simulink model "octocopter_control_flow"  (R2024a)
settings: Solver=FixedStepAuto  StartTime=0.0  StopTime=inf
model workspace (MAT data in the model file):
  Ixx_values = 1.545e-05
  Iyy_values = 0.00073574
  Izz_values = 0.00074861
  base_link_Ixx = 7.46
  base_link_Iyy = 1.52
  base_link_Izz = 8.88
  base_link_mass = 19.0939
  gps0_Ixx = 2.1733e-06
  gps0_Iyy = 2.1733e-06
  gps0_Izz = 1.8e-07
  gps0_mass = 0.01
  i = 8
  imu_link_Ixx = 1e-05
  imu_link_Iyy = 1e-05
  imu_link_Izz = 1e-05
  imu_link_mass = 0.015
  masses = 0.085251
  phi : object (value not decoded)
  rotors : object (value not decoded)
  theta : object (value not decoded)
  total_Ixx = 7.46
  total_Iyy = 1.53
  total_Izz = 8.89
  total_mass = 20
  total_rotor_Ixx = 0.0001236
  total_rotor_Iyy = 0.00588592
  total_rotor_Izz = 0.00598888
  total_rotor_masses = 0.682008
  u : object (value not decoded)
  v : object (value not decoded)
  w : object (value not decoded)
  x : object (value not decoded)
  y : object (value not decoded)
  z : object (value not decoded)
values from neighbouring files (symbols this model uses):
  err1Enable = 0    [drone_6dof.m]    (also in octocopter_model_for_agressive.m; octocopter_model_for_orbit.m)
  err2Enable = 0    [drone_6dof.m]    (also in octocopter_model_for_agressive.m; octocopter_model_for_orbit.m)
  err3Enable = 0    [drone_6dof.m]    (also in octocopter_model_for_agressive.m; octocopter_model_for_orbit.m)
  err4Enable = 0    [drone_6dof.m]    (also in octocopter_model_for_agressive.m; octocopter_model_for_orbit.m)
  err5Enable = 0    [drone_6dof.m]    (also in octocopter_model_for_agressive.m; octocopter_model_for_orbit.m)
  err6Enable = 0    [drone_6dof.m]    (also in octocopter_model_for_agressive.m; octocopter_model_for_orbit.m)
  err7Enable = 0    [drone_6dof.m]    (also in octocopter_model_for_agressive.m; octocopter_model_for_orbit.m)
  err8Enable = 0    [drone_6dof.m]    (also in octocopter_model_for_agressive.m; octocopter_model_for_orbit.m)
  EulerInt_initial = [0;0;0]    [drone_6dof.m]    (also in octocopter_model_for_agressive.m; octocopter_model_for_orbit.m)
  motorErr1Time = 0    [drone_6dof.m]    (also in octocopter_model_for_agressive.m; octocopter_model_for_orbit.m)
  motorErr2Time = 0    [drone_6dof.m]    (also in octocopter_model_for_agressive.m; octocopter_model_for_orbit.m)
  motorErr3Time = 0    [drone_6dof.m]    (also in octocopter_model_for_agressive.m; octocopter_model_for_orbit.m)
  motorErr4Time = 0    [drone_6dof.m]    (also in octocopter_model_for_agressive.m; octocopter_model_for_orbit.m)
  motorErr5Time = 0    [drone_6dof.m]    (also in octocopter_model_for_agressive.m; octocopter_model_for_orbit.m)
  motorErr6Time = 0    [drone_6dof.m]    (also in octocopter_model_for_agressive.m; octocopter_model_for_orbit.m)
  motorErr7Time = 0    [drone_6dof.m]    (also in octocopter_model_for_agressive.m; octocopter_model_for_orbit.m)
  motorErr8Time = 0    [drone_6dof.m]    (also in octocopter_model_for_agressive.m; octocopter_model_for_orbit.m)
  omegaInt_initial = [0;0;0]    [drone_6dof.m]    (also in octocopter_model_for_agressive.m; octocopter_model_for_orbit.m)
  PosInertialInt_initial = [0;0;0]    [drone_6dof.m]    (also in octocopter_model_for_agressive.m; octocopter_model_for_orbit.m)
  vbInt_initial = [0;0;0]    [drone_6dof.m]    (also in octocopter_model_for_agressive.m; octocopter_model_for_orbit.m)
undefined symbols (not defined in the file or in its folder): DiscIntNeverNeededParam, PID_x_D, PID_x_I, PID_x_N, PID_y_D, PID_y_I, PID_y_N, PID_z_D, PID_z_I, PID_z_N, rad, rotor_max_rad_per_s, rotor_min_rad_per_s, s
libraries: robotlib x15, slpidlib x10, aerolibconvert2 x10, cstblocks x7, simulink x6, sharedtransform x4, dspmathops x1, vrlib x1, sharedutil x1, simulink_extras x1
(part 2 of 2)

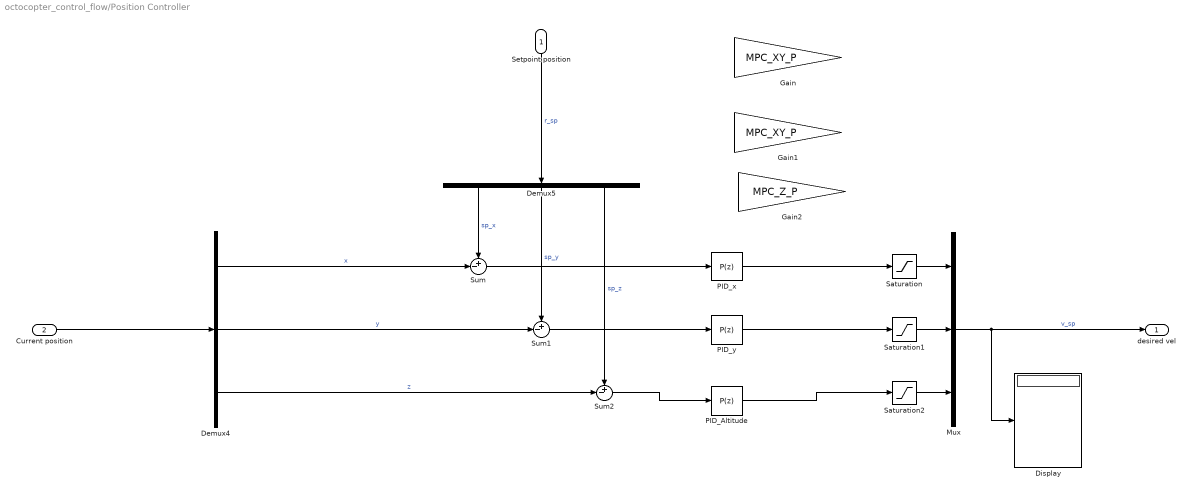
== system octocopter_control_flow/Position Controller ==
  Setpoint position : Inport
  Current position : Inport  Port=2
  Demux4 : Demux  Outputs=3
  Demux5 : Demux  Outputs=3
  Display : Display
  Gain : Gain  Gain=MPC_XY_P
  Gain1 : Gain  Gain=MPC_XY_P
  Gain2 : Gain  Gain=MPC_Z_P
  Mux : Mux  Inputs=3
  PID_Altitude : slpidlib/PID Controller  Controller=P  Form=Parallel  TimeDomain=Discrete-time  UseExternalTs=off  SampleTime=-1  IntegratorMethod=Backward Euler  FilterMethod=Forward Euler  ControllerParametersSource=internal  P=MPC_Z_P  I=PID_z_I  UseKiTs=off  D=PID_z_D  UseExternalDerivativeSource=off  N=PID_z_N  UseFilter=on  TunerSelectOption=Transfer Function Based (PID Tuner App)  InitialConditionSource=internal  InitialConditionForIntegrator=0  InitialConditionForFilter=0  DifferentiatorICPrevScaledInput=0  ExternalReset=level  TrackingMode=off  Kt=1  LimitOutput=on  SatLimitsSource=internal  UpperSaturationLimit=10  LowerSaturationLimit=-10  LinearizeAsGain=off  AntiWindupMode=clamping  Kb=1  LimitIntegrator=off  UpperIntegratorSaturationLimit=inf  LowerIntegratorSaturationLimit=-inf  POutMin=[]  POutMax=[]  IOutMin=[]  IOutMax=[]  DOutMin=[]  DOutMax=[]  NOutMin=[]  NOutMax=[]  SumOutMin=[]  SumOutMax=[]  SaturationOutMin=[]  SaturationOutMax=[]  PParamMin=[]  PParamMax=[]  IParamMin=[]  IParamMax=[]  DParamMin=[]  DParamMax=[]  NParamMin=[]  NParamMax=[]  KbParamMin=[]  KbParamMax=[]  KtParamMin=[]  KtParamMax=[]  KbOutMin=[]  KbOutMax=[]  KtOutMin=[]  KtOutMax=[]  IntegratorOutMin=[]  IntegratorOutMax=[]  FilterOutMin=[]  FilterOutMax=[]  SumI1OutMin=[]  SumI1OutMax=[]  SumI2OutMin=[]  SumI2OutMax=[]  SumI3OutMin=[]  SumI3OutMax=[]  SumI4OutMin=[]  SumI4OutMax=[]  SumDOutMin=[]  SumDOutMax=[]  DifferentiatorOutMin=[]  DifferentiatorOutMax=[]  FilterDiffOutCoefMin=[]  FilterDiffOutCoefMax=[]  ReciprocalOutMin=[]  ReciprocalOutMax=[]  SumDenOutMin=[]  SumDenOutMax=[]  SumNumOutMin=[]  SumNumOutMax=[]  DivideOutMin=[]  DivideOutMax=[]  UdiffTsProdOutMin=[]  UdiffTsProdOutMax=[]  NTsProdOutMin=[]  NTsProdOutMax=[]  UintegralTsProdOutMin=[]  UintegralTsProdOutMax=[]  UngainTsProdOutMin=[]  UngainTsProdOutMax=[]  ClampingZeroOutDataTypeStr=Inherit: Inherit via back propagation  ClampingZeroOutMin=[]  ClampingZeroOutMax=[]  FilterDenConstantOutDataTypeStr=Inherit: Inherit via back propagation  FilterDenConstantOutMin=[]  FilterDenConstantOutMax=[]  PCopyOutDataTypeStr=Inherit: Inherit via back propagation  PCopyOutMin=[]  PCopyOutMax=[]  NCopyOutDataTypeStr=Inherit: Inherit via back propagation  NCopyOutMin=[]  NCopyOutMax=[]  IntegratorContinuousStateAttributes=''  IntegratorStateMustResolveToSignalObject=off  IntegratorRTWStateStorageClass=Auto  FilterContinuousStateAttributes=''  FilterStateMustResolveToSignalObject=off  FilterRTWStateStorageClass=Auto  ParallelPVariant=InternalParameters  IdealPVariant=Disabled  IVariant=Disabled  DVariant=Disabled  IntegratorVariant=Disabled  SatVariant=Enabled  AWVariant=Disabled  PCopyVariant=Disabled  TRVariant=Disabled  FdbkBlocksVariant=Forward  IdealPFdbkVariant=Disabled  SatFdbkVariant=Disabled  DerivativeFilterVariant=Disabled  NVariant=Disabled  NCopyVariant=Disabled_SignalSpec  FilterICVariant=Disabled  IntegratorICVariant=Disabled  ExternalResetVariant=Disabled  TRSumVariant=Passthrough  SumFdbkVariant=Disabled  SumVariant=Passthrough_P  TsampFilterVariant=InternalTs  TsampNgainVariant=Passthrough  TsampIntegralVariant=Disabled_SignalSpec  ExternalSaturationOutDataTypeStr=Inherit: Same as second input  DerivativeSourceVariant=Disabled
  PID_x : slpidlib/PID Controller  Controller=P  Form=Parallel  TimeDomain=Discrete-time  UseExternalTs=off  SampleTime=-1  IntegratorMethod=Forward Euler  FilterMethod=Forward Euler  ControllerParametersSource=internal  P=MPC_XY_P  I=PID_x_I  UseKiTs=off  D=PID_x_D  UseExternalDerivativeSource=off  N=PID_x_N  UseFilter=on  TunerSelectOption=Transfer Function Based (PID Tuner App)  InitialConditionSource=internal  InitialConditionForIntegrator=0  InitialConditionForFilter=0  DifferentiatorICPrevScaledInput=0  ExternalReset=level  TrackingMode=off  Kt=1  LimitOutput=on  SatLimitsSource=internal  UpperSaturationLimit=20  LowerSaturationLimit=-20  LinearizeAsGain=off  AntiWindupMode=clamping  Kb=1  LimitIntegrator=off  UpperIntegratorSaturationLimit=inf  LowerIntegratorSaturationLimit=-inf  POutMin=[]  POutMax=[]  IOutMin=[]  IOutMax=[]  DOutMin=[]  DOutMax=[]  NOutMin=[]  NOutMax=[]  SumOutMin=[]  SumOutMax=[]  SaturationOutMin=[]  SaturationOutMax=[]  PParamMin=[]  PParamMax=[]  IParamMin=[]  IParamMax=[]  DParamMin=[]  DParamMax=[]  NParamMin=[]  NParamMax=[]  KbParamMin=[]  KbParamMax=[]  KtParamMin=[]  KtParamMax=[]  KbOutMin=[]  KbOutMax=[]  KtOutMin=[]  KtOutMax=[]  IntegratorOutMin=[]  IntegratorOutMax=[]  FilterOutMin=[]  FilterOutMax=[]  SumI1OutMin=[]  SumI1OutMax=[]  SumI2OutMin=[]  SumI2OutMax=[]  SumI3OutMin=[]  SumI3OutMax=[]  SumI4OutMin=[]  SumI4OutMax=[]  SumDOutMin=[]  SumDOutMax=[]  DifferentiatorOutMin=[]  DifferentiatorOutMax=[]  FilterDiffOutCoefMin=[]  FilterDiffOutCoefMax=[]  ReciprocalOutMin=[]  ReciprocalOutMax=[]  SumDenOutMin=[]  SumDenOutMax=[]  SumNumOutMin=[]  SumNumOutMax=[]  DivideOutMin=[]  DivideOutMax=[]  UdiffTsProdOutMin=[]  UdiffTsProdOutMax=[]  NTsProdOutMin=[]  NTsProdOutMax=[]  UintegralTsProdOutMin=[]  UintegralTsProdOutMax=[]  UngainTsProdOutMin=[]  UngainTsProdOutMax=[]  ClampingZeroOutDataTypeStr=Inherit: Inherit via back propagation  ClampingZeroOutMin=[]  ClampingZeroOutMax=[]  FilterDenConstantOutDataTypeStr=Inherit: Inherit via back propagation  FilterDenConstantOutMin=[]  FilterDenConstantOutMax=[]  PCopyOutDataTypeStr=Inherit: Inherit via back propagation  PCopyOutMin=[]  PCopyOutMax=[]  NCopyOutDataTypeStr=Inherit: Inherit via back propagation  NCopyOutMin=[]  NCopyOutMax=[]  IntegratorContinuousStateAttributes=''  IntegratorStateMustResolveToSignalObject=off  IntegratorRTWStateStorageClass=Auto  FilterContinuousStateAttributes=''  FilterStateMustResolveToSignalObject=off  FilterRTWStateStorageClass=Auto  ParallelPVariant=InternalParameters  IdealPVariant=Disabled  IVariant=Disabled  DVariant=Disabled  IntegratorVariant=Disabled  SatVariant=Enabled  AWVariant=Disabled  PCopyVariant=Disabled  TRVariant=Disabled  FdbkBlocksVariant=Forward  IdealPFdbkVariant=Disabled  SatFdbkVariant=Disabled  DerivativeFilterVariant=Disabled  NVariant=Disabled  NCopyVariant=Disabled_SignalSpec  FilterICVariant=Disabled  IntegratorICVariant=Disabled  ExternalResetVariant=Disabled  TRSumVariant=Passthrough  SumFdbkVariant=Disabled  SumVariant=Passthrough_P  TsampFilterVariant=InternalTs  TsampNgainVariant=Passthrough  TsampIntegralVariant=Disabled_SignalSpec  ExternalSaturationOutDataTypeStr=Inherit: Same as second input  DerivativeSourceVariant=Disabled
  PID_y : slpidlib/PID Controller  Controller=P  Form=Parallel  TimeDomain=Discrete-time  UseExternalTs=off  SampleTime=-1  IntegratorMethod=Forward Euler  FilterMethod=Forward Euler  ControllerParametersSource=internal  P=MPC_XY_P  I=PID_y_I  UseKiTs=off  D=PID_y_D  UseExternalDerivativeSource=off  N=PID_y_N  UseFilter=on  TunerSelectOption=Transfer Function Based (PID Tuner App)  InitialConditionSource=internal  InitialConditionForIntegrator=0  InitialConditionForFilter=0  DifferentiatorICPrevScaledInput=0  ExternalReset=level  TrackingMode=off  Kt=1  LimitOutput=on  SatLimitsSource=internal  UpperSaturationLimit=20  LowerSaturationLimit=-20  LinearizeAsGain=off  AntiWindupMode=clamping  Kb=1  LimitIntegrator=off  UpperIntegratorSaturationLimit=inf  LowerIntegratorSaturationLimit=-inf  POutMin=[]  POutMax=[]  IOutMin=[]  IOutMax=[]  DOutMin=[]  DOutMax=[]  NOutMin=[]  NOutMax=[]  SumOutMin=[]  SumOutMax=[]  SaturationOutMin=[]  SaturationOutMax=[]  PParamMin=[]  PParamMax=[]  IParamMin=[]  IParamMax=[]  DParamMin=[]  DParamMax=[]  NParamMin=[]  NParamMax=[]  KbParamMin=[]  KbParamMax=[]  KtParamMin=[]  KtParamMax=[]  KbOutMin=[]  KbOutMax=[]  KtOutMin=[]  KtOutMax=[]  IntegratorOutMin=[]  IntegratorOutMax=[]  FilterOutMin=[]  FilterOutMax=[]  SumI1OutMin=[]  SumI1OutMax=[]  SumI2OutMin=[]  SumI2OutMax=[]  SumI3OutMin=[]  SumI3OutMax=[]  SumI4OutMin=[]  SumI4OutMax=[]  SumDOutMin=[]  SumDOutMax=[]  DifferentiatorOutMin=[]  DifferentiatorOutMax=[]  FilterDiffOutCoefMin=[]  FilterDiffOutCoefMax=[]  ReciprocalOutMin=[]  ReciprocalOutMax=[]  SumDenOutMin=[]  SumDenOutMax=[]  SumNumOutMin=[]  SumNumOutMax=[]  DivideOutMin=[]  DivideOutMax=[]  UdiffTsProdOutMin=[]  UdiffTsProdOutMax=[]  NTsProdOutMin=[]  NTsProdOutMax=[]  UintegralTsProdOutMin=[]  UintegralTsProdOutMax=[]  UngainTsProdOutMin=[]  UngainTsProdOutMax=[]  ClampingZeroOutDataTypeStr=Inherit: Inherit via back propagation  ClampingZeroOutMin=[]  ClampingZeroOutMax=[]  FilterDenConstantOutDataTypeStr=Inherit: Inherit via back propagation  FilterDenConstantOutMin=[]  FilterDenConstantOutMax=[]  PCopyOutDataTypeStr=Inherit: Inherit via back propagation  PCopyOutMin=[]  PCopyOutMax=[]  NCopyOutDataTypeStr=Inherit: Inherit via back propagation  NCopyOutMin=[]  NCopyOutMax=[]  IntegratorContinuousStateAttributes=''  IntegratorStateMustResolveToSignalObject=off  IntegratorRTWStateStorageClass=Auto  FilterContinuousStateAttributes=''  FilterStateMustResolveToSignalObject=off  FilterRTWStateStorageClass=Auto  ParallelPVariant=InternalParameters  IdealPVariant=Disabled  IVariant=Disabled  DVariant=Disabled  IntegratorVariant=Disabled  SatVariant=Enabled  AWVariant=Disabled  PCopyVariant=Disabled  TRVariant=Disabled  FdbkBlocksVariant=Forward  IdealPFdbkVariant=Disabled  SatFdbkVariant=Disabled  DerivativeFilterVariant=Disabled  NVariant=Disabled  NCopyVariant=Disabled_SignalSpec  FilterICVariant=Disabled  IntegratorICVariant=Disabled  ExternalResetVariant=Disabled  TRSumVariant=Passthrough  SumFdbkVariant=Disabled  SumVariant=Passthrough_P  TsampFilterVariant=InternalTs  TsampNgainVariant=Passthrough  TsampIntegralVariant=Disabled_SignalSpec  ExternalSaturationOutDataTypeStr=Inherit: Same as second input  DerivativeSourceVariant=Disabled
  Saturation : Saturate  UpperLimit=MPC_XY_VEL_ALL  LowerLimit=-MPC_XY_VEL_ALL
  Saturation1 : Saturate  UpperLimit=MPC_XY_VEL_ALL  LowerLimit=-MPC_XY_VEL_ALL
  Saturation2 : Saturate  UpperLimit=1  LowerLimit=-1
  Sum : Sum  Inputs=+-|
  Sum1 : Sum  Inputs=+-|
  Sum2 : Sum  Inputs=+-|
  desired vel : Outport
  wires:
  Sum2/1 -> PID_Altitude/1
  Demux4/3 -> Sum2/2  "z"
  Current position/1 -> Demux4/1
  Saturation1/1 -> Mux/2
  Demux5/2 -> Sum1/1  "sp_y"
  Sum/1 -> PID_x/1
  Demux4/1 -> Sum/2  "x"
  PID_y/1 -> Saturation1/1
  Mux/1 -> desired vel/1, Display/1  "v_sp"
  Saturation2/1 -> Mux/3
  PID_x/1 -> Saturation/1
  PID_Altitude/1 -> Saturation2/1
  Demux5/1 -> Sum/1  "sp_x"
  Demux4/2 -> Sum1/2  "y"
  Demux5/3 -> Sum2/1  "sp_z"
  Saturation/1 -> Mux/1
  Setpoint position/1 -> Demux5/1  "r_sp"
  Sum1/1 -> PID_y/1

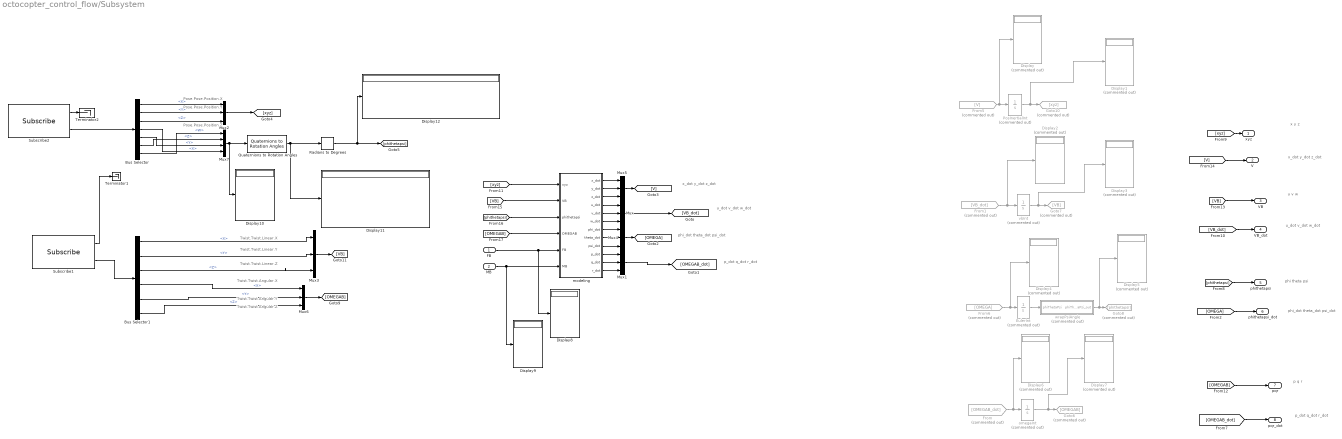
== system octocopter_control_flow/Subsystem ==
  note: Pose.Pose.Position.X
  note: x
      | y
      | z
  note: x_dot
      | y_dot
      | z_dot
  note: phi_dot
      | theta_dot
      | psi_dot
  note: phi
      | theta
      | psi
  note: p_dot
      | q_dot
      | r_dot
  note: p
      | q
      | r
  note: u
      | v
      | w
  note: u_dot
      | v_dot
      | w_dot
  note: x_dot
      | y_dot
      | z_dot
  note: u_dot
      | v_dot
      | w_dot
  note: phi_dot
      | theta_dot
      | psi_dot
  note: p_dot
      | q_dot
      | r_dot
  note: Pose.Pose.Position.Y
  note: Pose.Pose.Position.Z
  note: Twist.Twist.Linear.X
  note: Twist.Twist.Linear.Y
  note: Twist.Twist.Linear.Z
  note: Twist.Twist.Angular.X
  note: Twist.Twist.Angular.Y
  note: Twist.Twist.Angular.Z
  FB : Inport
  MB : Inport  Port=2
  Bus Selector : BusSelector  OutputSignals=Pose.Pose.Position.X,Pose.Pose.Position.Y,Pose.Pose.Position.Z,Pose.Pose.Orientation.X,Pose.Pose.Orientation.Y,Pose.Pose.Orientation.Z,Pose.Pose.Orientation.W
  Bus Selector1 : BusSelector  OutputSignals=Twist.Twist.Linear.X,Twist.Twist.Linear.Y,Twist.Twist.Linear.Z,Twist.Twist.Angular.X,Twist.Twist.Angular.Y,Twist.Twist.Angular.Z
  Display{,1..7} (8 alike) : Display  Commented=on
  Display{8..12} (5 alike) : Display
  EulerInt : Integrator  Commented=on  InitialCondition=EulerInt_initial
  From : From  Commented=on  GotoTag=OMEGAB_dot
  From1 : From  Commented=on  GotoTag=VB_dot
  From5 : From  Commented=on  GotoTag=V
  From6 : From  Commented=on  GotoTag=OMEGA
  Goto10 : Goto  Commented=on  GotoTag=xyz
  Goto6 : Goto  Commented=on  GotoTag=OMEGAB
  Goto7 : Goto  Commented=on  GotoTag=VB
  Goto8 : Goto  Commented=on  GotoTag=phithetapsi
  Mux{,1..6} (7 alike) : Mux  Inputs=3
  Mux7 : Mux
  PosInertialInt : Integrator  Commented=on  InitialCondition=PosInertialInt_initial
  Quaternions to Rotation Angles : sharedtransform/Quaternions to Rotation Angles  rotationOrder=ZYX  aMode=aMode
  Radians to Degrees : simulink_extras/Transformations/Radians to Degrees
  Subscribe1 : robotlib/Subscribe  topicSource=Select from ROS network  topic=/mavros/local_position/odom  messageType=nav_msgs/Odometry  SampleTime=-1  legacyBusStruct=off  messageQueueLength=1
  Subscribe2 : robotlib/Subscribe  topicSource=Select from ROS network  topic=/mavros/global_position/local  messageType=nav_msgs/Odometry  SampleTime=-1  legacyBusStruct=off  messageQueueLength=1
  Terminator1 : Terminator
  Terminator2 : Terminator
  modeling : MATLAB Function  TreatAsAtomicUnit=on
  omegaInt : Integrator  Commented=on  InitialCondition=omegaInt_initial  UpperSaturationLimit=rotor_max_rad_per_s  LowerSaturationLimit=rotor_min_rad_per_s
  vbInt : Integrator  Commented=on  InitialCondition=vbInt_initial
  wrapPsiAngle : Subsystem  Commented=on
  xyz : Outport
  V : Outport  Port=2
  VB : Outport  Port=3
  VB_dot : Outport  Port=4
  phithetapsi : Outport  Port=5
  phithetapsi_dot : Outport  Port=6
  pqr : Outport  Port=7
  pqr_dot : Outport  Port=8
  wires:
  From1/1 -> Display2/1, vbInt/1
  From5/1 -> Display/1, PosInertialInt/1
  EulerInt/1 -> wrapPsiAngle/1(phiThetaPsi)
  Mux1/1 -> [OMEGAB_dot]
  Mux4/1 -> [OMEGA]
  Mux/1 -> [VB_dot]
  PosInertialInt/1 -> Display1/1, Goto10/1
  Mux5/1 -> [V]
  omegaInt/1 -> Display7/1, Goto6/1
  modeling/11(q_dot) -> Mux1/2
  From6/1 -> Display4/1, EulerInt/1
  modeling/6(w_dot) -> Mux/3
  [V] -> V/1
  [xyz] -> xyz/1
  From/1 -> Display6/1, omegaInt/1
  modeling/3(z_dot) -> Mux5/3
  [phithetapsi] -> phithetapsi/1
  wrapPsiAngle/1(phiThetaPsi_out) -> Display5/1, Goto8/1
  modeling/4(u_dot) -> Mux/1
  modeling/8(theta_dot) -> Mux4/2
  modeling/5(v_dot) -> Mux/2
  modeling/12(r_dot) -> Mux1/3
  modeling/9(psi_dot) -> Mux4/3
  vbInt/1 -> Display3/1, Goto7/1
  modeling/7(phi_dot) -> Mux4/1
  modeling/2(y_dot) -> Mux5/2
  modeling/10(p_dot) -> Mux1/1
  modeling/1(x_dot) -> Mux5/1
  [OMEGA] -> phithetapsi_dot/1
  [OMEGAB_dot] -> pqr_dot/1
  [OMEGAB] -> pqr/1
  [VB_dot] -> VB_dot/1
  [VB] -> VB/1
  FB/1 -> Display8/1, modeling/5(FB)
  MB/1 -> Display9/1, modeling/6(MB)
  [OMEGAB] -> modeling/4(OMEGAB)
  [phithetapsi] -> modeling/3(phithetapsi)
  [VB] -> modeling/2(VB)
  [xyz] -> modeling/1(xyz)
  Bus Selector1/2 -> Mux3/2  "<Y>"
  Subscribe1/2 -> Bus Selector1/1
  Bus Selector1/4 -> Mux6/1  "<X>"
  Bus Selector1/1 -> Mux3/1  "<X>"
  Subscribe1/1 -> Terminator1/1
  Bus Selector1/3 -> Mux3/3  "<Z>"
  Bus Selector1/6 -> Mux6/3  "<Z>"
  Bus Selector1/5 -> Mux6/2  "<Y>"
  Mux2/1 -> [xyz]
  Mux6/1 -> [OMEGAB]
  Mux3/1 -> [VB]
  Subscribe2/2 -> Bus Selector/1
  Subscribe2/1 -> Terminator2/1
  Bus Selector/2 -> Mux2/2  "<Y>"
  Bus Selector/1 -> Mux2/1  "<X>"
  Bus Selector/3 -> Mux2/3  "<Z>"
  Mux7/1 -> Display10/1, Quaternions to Rotation Angles/1
  Quaternions to Rotation Angles/1 -> Display11/1, Radians to Degrees/1
  Bus Selector/7 -> Mux7/1  "<W>"
  Bus Selector/4 -> Mux7/4  "<X>"
  Bus Selector/5 -> Mux7/3  "<Y>"
  Bus Selector/6 -> Mux7/2  "<Z>"
  Radians to Degrees/1 -> Display12/1, [phithetapsi]

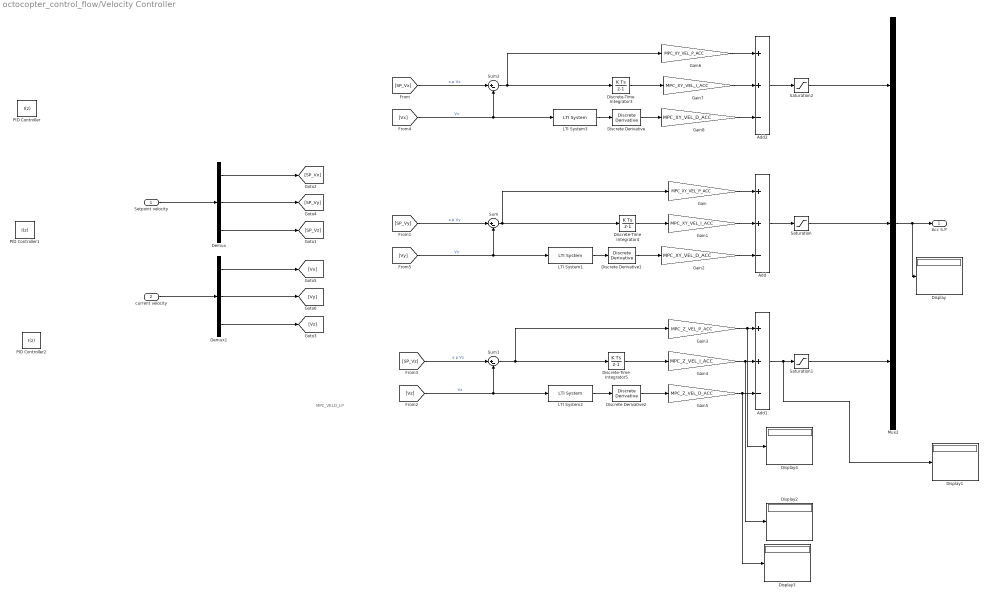
== system octocopter_control_flow/Velocity Controller ==
  note: MPC_VELD_LP
  Setpoint velocity : Inport
  current velocity : Inport  Port=2
  Add : Sum  Inputs=++-
  Add1 : Sum  Inputs=++-
  Add2 : Sum  Inputs=++-
  Demux : Demux  Outputs=3
  Demux1 : Demux  Outputs=3
  Discrete Derivative : simulink/Discrete/Discrete Derivative  gainval=1.0  ICPrevScaledInput=0.0  OutMin=[]  OutMax=[]  OutDataType=fixdt(1, 16)  OutScaling=2^-10  DoSatur=off
  Discrete Derivative1 : simulink/Discrete/Discrete Derivative  gainval=1.0  ICPrevScaledInput=0.0  OutMin=[]  OutMax=[]  OutDataType=fixdt(1, 16)  OutScaling=2^-10  DoSatur=off
  Discrete Derivative2 : simulink/Discrete/Discrete Derivative  gainval=1.0  ICPrevScaledInput=0.0  OutMin=[]  OutMax=[]  OutDataType=fixdt(1, 16)  OutScaling=2^-10  DoSatur=off
  Discrete-Time Integrator3 : DiscreteIntegrator  SampleTime=1/100  ICPrevOutput=DiscIntNeverNeededParam  ICPrevScaledInput=DiscIntNeverNeededParam
  Discrete-Time Integrator4 : DiscreteIntegrator  SampleTime=1/100  ICPrevOutput=DiscIntNeverNeededParam  ICPrevScaledInput=DiscIntNeverNeededParam
  Discrete-Time Integrator5 : DiscreteIntegrator  SampleTime=1/100  ICPrevOutput=DiscIntNeverNeededParam  ICPrevScaledInput=DiscIntNeverNeededParam
  Display{,1..4} (5 alike) : Display
  Gain : Gain  Gain=MPC_XY_VEL_P_ACC
  Gain1 : Gain  Gain=MPC_XY_VEL_I_ACC
  Gain2 : Gain  Gain=MPC_XY_VEL_D_ACC
  Gain3 : Gain  Gain=MPC_Z_VEL_P_ACC
  Gain4 : Gain  Gain=MPC_Z_VEL_I_ACC
  Gain5 : Gain  Gain=MPC_Z_VEL_D_ACC
  Gain6 : Gain  Gain=MPC_XY_VEL_P_ACC
  Gain7 : Gain  Gain=MPC_XY_VEL_I_ACC
  Gain8 : Gain  Gain=MPC_XY_VEL_D_ACC
  LTI System1 : cstblocks/LTI System  sys=c2d(tf(1,[MPC_VELD_LP 1]),1/100)  IC=[]  PadeOrder=0
  LTI System2 : cstblocks/LTI System  sys=c2d(tf(1,[MPC_VELD_LP 1]),1/100)  IC=[]  PadeOrder=0
  LTI System3 : cstblocks/LTI System  sys=c2d(tf(1,[MPC_VELD_LP 1]),1/100)  IC=[]  PadeOrder=0
  Mux2 : Mux  Inputs=3
  PID Controller : slpidlib/PID Controller  Controller=I  Form=Parallel  TimeDomain=Discrete-time  UseExternalTs=off  SampleTime=-1  IntegratorMethod=Forward Euler  FilterMethod=Forward Euler  ControllerParametersSource=internal  P=MPC_XY_VEL_P_ACC  I=MPC_XY_VEL_I_ACC  UseKiTs=off  D=0  UseExternalDerivativeSource=off  N=100  UseFilter=on  TunerSelectOption=Transfer Function Based (PID Tuner App)  InitialConditionSource=internal  InitialConditionForIntegrator=0  InitialConditionForFilter=0  DifferentiatorICPrevScaledInput=0  ExternalReset=none  TrackingMode=off  Kt=1  LimitOutput=on  SatLimitsSource=internal  UpperSaturationLimit=inf  LowerSaturationLimit=-inf  LinearizeAsGain=on  AntiWindupMode=clamping  Kb=1  LimitIntegrator=off  UpperIntegratorSaturationLimit=inf  LowerIntegratorSaturationLimit=-inf  POutMin=[]  POutMax=[]  IOutMin=[]  IOutMax=[]  DOutMin=[]  DOutMax=[]  NOutMin=[]  NOutMax=[]  SumOutMin=[]  SumOutMax=[]  SaturationOutMin=[]  SaturationOutMax=[]  PParamMin=[]  PParamMax=[]  IParamMin=[]  IParamMax=[]  DParamMin=[]  DParamMax=[]  NParamMin=[]  NParamMax=[]  KbParamMin=[]  KbParamMax=[]  KtParamMin=[]  KtParamMax=[]  KbOutMin=[]  KbOutMax=[]  KtOutMin=[]  KtOutMax=[]  IntegratorOutMin=[]  IntegratorOutMax=[]  FilterOutMin=[]  FilterOutMax=[]  SumI1OutMin=[]  SumI1OutMax=[]  SumI2OutMin=[]  SumI2OutMax=[]  SumI3OutMin=[]  SumI3OutMax=[]  SumI4OutMin=[]  SumI4OutMax=[]  SumDOutMin=[]  SumDOutMax=[]  DifferentiatorOutMin=[]  DifferentiatorOutMax=[]  FilterDiffOutCoefMin=[]  FilterDiffOutCoefMax=[]  ReciprocalOutMin=[]  ReciprocalOutMax=[]  SumDenOutMin=[]  SumDenOutMax=[]  SumNumOutMin=[]  SumNumOutMax=[]  DivideOutMin=[]  DivideOutMax=[]  UdiffTsProdOutMin=[]  UdiffTsProdOutMax=[]  NTsProdOutMin=[]  NTsProdOutMax=[]  UintegralTsProdOutMin=[]  UintegralTsProdOutMax=[]  UngainTsProdOutMin=[]  UngainTsProdOutMax=[]  ClampingZeroOutDataTypeStr=Inherit: Inherit via back propagation  ClampingZeroOutMin=[]  ClampingZeroOutMax=[]  FilterDenConstantOutDataTypeStr=Inherit: Inherit via back propagation  FilterDenConstantOutMin=[]  FilterDenConstantOutMax=[]  PCopyOutDataTypeStr=Inherit: Inherit via back propagation  PCopyOutMin=[]  PCopyOutMax=[]  NCopyOutDataTypeStr=Inherit: Inherit via back propagation  NCopyOutMin=[]  NCopyOutMax=[]  IntegratorContinuousStateAttributes=''  IntegratorStateMustResolveToSignalObject=off  IntegratorRTWStateStorageClass=Auto  FilterContinuousStateAttributes=''  FilterStateMustResolveToSignalObject=off  FilterRTWStateStorageClass=Auto  ParallelPVariant=Disabled  IdealPVariant=Disabled  IVariant=InternalParameters  DVariant=Disabled  IntegratorVariant=Discrete  SatVariant=Enabled  AWVariant=DiscClampingParallel  PCopyVariant=Disabled  TRVariant=Disabled  FdbkBlocksVariant=Forward  IdealPFdbkVariant=Disabled  SatFdbkVariant=Disabled  DerivativeFilterVariant=Disabled  NVariant=Disabled  NCopyVariant=Disabled_SignalSpec  FilterICVariant=Disabled  IntegratorICVariant=InternalICs  ExternalResetVariant=Disabled  TRSumVariant=Passthrough  SumFdbkVariant=Disabled  SumVariant=Passthrough_I  TsampFilterVariant=InternalTs  TsampNgainVariant=Passthrough  TsampIntegralVariant=Disabled_SignalSpec  ExternalSaturationOutDataTypeStr=Inherit: Same as second input  DerivativeSourceVariant=Disabled
  PID Controller1 : slpidlib/PID Controller  Controller=I  Form=Parallel  TimeDomain=Discrete-time  UseExternalTs=off  SampleTime=-1  IntegratorMethod=Forward Euler  FilterMethod=Forward Euler  ControllerParametersSource=internal  P=MPC_XY_VEL_P_ACC  I=MPC_XY_VEL_I_ACC  UseKiTs=off  D=0  UseExternalDerivativeSource=off  N=100  UseFilter=on  TunerSelectOption=Transfer Function Based (PID Tuner App)  InitialConditionSource=internal  InitialConditionForIntegrator=0  InitialConditionForFilter=0  DifferentiatorICPrevScaledInput=0  ExternalReset=none  TrackingMode=off  Kt=1  LimitOutput=on  SatLimitsSource=internal  UpperSaturationLimit=inf  LowerSaturationLimit=-inf  LinearizeAsGain=on  AntiWindupMode=clamping  Kb=1  LimitIntegrator=off  UpperIntegratorSaturationLimit=inf  LowerIntegratorSaturationLimit=-inf  POutMin=[]  POutMax=[]  IOutMin=[]  IOutMax=[]  DOutMin=[]  DOutMax=[]  NOutMin=[]  NOutMax=[]  SumOutMin=[]  SumOutMax=[]  SaturationOutMin=[]  SaturationOutMax=[]  PParamMin=[]  PParamMax=[]  IParamMin=[]  IParamMax=[]  DParamMin=[]  DParamMax=[]  NParamMin=[]  NParamMax=[]  KbParamMin=[]  KbParamMax=[]  KtParamMin=[]  KtParamMax=[]  KbOutMin=[]  KbOutMax=[]  KtOutMin=[]  KtOutMax=[]  IntegratorOutMin=[]  IntegratorOutMax=[]  FilterOutMin=[]  FilterOutMax=[]  SumI1OutMin=[]  SumI1OutMax=[]  SumI2OutMin=[]  SumI2OutMax=[]  SumI3OutMin=[]  SumI3OutMax=[]  SumI4OutMin=[]  SumI4OutMax=[]  SumDOutMin=[]  SumDOutMax=[]  DifferentiatorOutMin=[]  DifferentiatorOutMax=[]  FilterDiffOutCoefMin=[]  FilterDiffOutCoefMax=[]  ReciprocalOutMin=[]  ReciprocalOutMax=[]  SumDenOutMin=[]  SumDenOutMax=[]  SumNumOutMin=[]  SumNumOutMax=[]  DivideOutMin=[]  DivideOutMax=[]  UdiffTsProdOutMin=[]  UdiffTsProdOutMax=[]  NTsProdOutMin=[]  NTsProdOutMax=[]  UintegralTsProdOutMin=[]  UintegralTsProdOutMax=[]  UngainTsProdOutMin=[]  UngainTsProdOutMax=[]  ClampingZeroOutDataTypeStr=Inherit: Inherit via back propagation  ClampingZeroOutMin=[]  ClampingZeroOutMax=[]  FilterDenConstantOutDataTypeStr=Inherit: Inherit via back propagation  FilterDenConstantOutMin=[]  FilterDenConstantOutMax=[]  PCopyOutDataTypeStr=Inherit: Inherit via back propagation  PCopyOutMin=[]  PCopyOutMax=[]  NCopyOutDataTypeStr=Inherit: Inherit via back propagation  NCopyOutMin=[]  NCopyOutMax=[]  IntegratorContinuousStateAttributes=''  IntegratorStateMustResolveToSignalObject=off  IntegratorRTWStateStorageClass=Auto  FilterContinuousStateAttributes=''  FilterStateMustResolveToSignalObject=off  FilterRTWStateStorageClass=Auto  ParallelPVariant=Disabled  IdealPVariant=Disabled  IVariant=InternalParameters  DVariant=Disabled  IntegratorVariant=Discrete  SatVariant=Enabled  AWVariant=DiscClampingParallel  PCopyVariant=Disabled  TRVariant=Disabled  FdbkBlocksVariant=Forward  IdealPFdbkVariant=Disabled  SatFdbkVariant=Disabled  DerivativeFilterVariant=Disabled  NVariant=Disabled  NCopyVariant=Disabled_SignalSpec  FilterICVariant=Disabled  IntegratorICVariant=InternalICs  ExternalResetVariant=Disabled  TRSumVariant=Passthrough  SumFdbkVariant=Disabled  SumVariant=Passthrough_I  TsampFilterVariant=InternalTs  TsampNgainVariant=Passthrough  TsampIntegralVariant=Disabled_SignalSpec  ExternalSaturationOutDataTypeStr=Inherit: Same as second input  DerivativeSourceVariant=Disabled
  PID Controller2 : slpidlib/PID Controller  Controller=I  Form=Parallel  TimeDomain=Discrete-time  UseExternalTs=off  SampleTime=-1  IntegratorMethod=Forward Euler  FilterMethod=Forward Euler  ControllerParametersSource=internal  P=MPC_XY_VEL_P_ACC  I=MPC_Z_VEL_I_ACC  UseKiTs=off  D=0  UseExternalDerivativeSource=off  N=100  UseFilter=on  TunerSelectOption=Transfer Function Based (PID Tuner App)  InitialConditionSource=internal  InitialConditionForIntegrator=0  InitialConditionForFilter=0  DifferentiatorICPrevScaledInput=0  ExternalReset=none  TrackingMode=off  Kt=1  LimitOutput=on  SatLimitsSource=internal  UpperSaturationLimit=inf  LowerSaturationLimit=-inf  LinearizeAsGain=on  AntiWindupMode=clamping  Kb=1  LimitIntegrator=off  UpperIntegratorSaturationLimit=inf  LowerIntegratorSaturationLimit=-inf  POutMin=[]  POutMax=[]  IOutMin=[]  IOutMax=[]  DOutMin=[]  DOutMax=[]  NOutMin=[]  NOutMax=[]  SumOutMin=[]  SumOutMax=[]  SaturationOutMin=[]  SaturationOutMax=[]  PParamMin=[]  PParamMax=[]  IParamMin=[]  IParamMax=[]  DParamMin=[]  DParamMax=[]  NParamMin=[]  NParamMax=[]  KbParamMin=[]  KbParamMax=[]  KtParamMin=[]  KtParamMax=[]  KbOutMin=[]  KbOutMax=[]  KtOutMin=[]  KtOutMax=[]  IntegratorOutMin=[]  IntegratorOutMax=[]  FilterOutMin=[]  FilterOutMax=[]  SumI1OutMin=[]  SumI1OutMax=[]  SumI2OutMin=[]  SumI2OutMax=[]  SumI3OutMin=[]  SumI3OutMax=[]  SumI4OutMin=[]  SumI4OutMax=[]  SumDOutMin=[]  SumDOutMax=[]  DifferentiatorOutMin=[]  DifferentiatorOutMax=[]  FilterDiffOutCoefMin=[]  FilterDiffOutCoefMax=[]  ReciprocalOutMin=[]  ReciprocalOutMax=[]  SumDenOutMin=[]  SumDenOutMax=[]  SumNumOutMin=[]  SumNumOutMax=[]  DivideOutMin=[]  DivideOutMax=[]  UdiffTsProdOutMin=[]  UdiffTsProdOutMax=[]  NTsProdOutMin=[]  NTsProdOutMax=[]  UintegralTsProdOutMin=[]  UintegralTsProdOutMax=[]  UngainTsProdOutMin=[]  UngainTsProdOutMax=[]  ClampingZeroOutDataTypeStr=Inherit: Inherit via back propagation  ClampingZeroOutMin=[]  ClampingZeroOutMax=[]  FilterDenConstantOutDataTypeStr=Inherit: Inherit via back propagation  FilterDenConstantOutMin=[]  FilterDenConstantOutMax=[]  PCopyOutDataTypeStr=Inherit: Inherit via back propagation  PCopyOutMin=[]  PCopyOutMax=[]  NCopyOutDataTypeStr=Inherit: Inherit via back propagation  NCopyOutMin=[]  NCopyOutMax=[]  IntegratorContinuousStateAttributes=''  IntegratorStateMustResolveToSignalObject=off  IntegratorRTWStateStorageClass=Auto  FilterContinuousStateAttributes=''  FilterStateMustResolveToSignalObject=off  FilterRTWStateStorageClass=Auto  ParallelPVariant=Disabled  IdealPVariant=Disabled  IVariant=InternalParameters  DVariant=Disabled  IntegratorVariant=Discrete  SatVariant=Enabled  AWVariant=DiscClampingParallel  PCopyVariant=Disabled  TRVariant=Disabled  FdbkBlocksVariant=Forward  IdealPFdbkVariant=Disabled  SatFdbkVariant=Disabled  DerivativeFilterVariant=Disabled  NVariant=Disabled  NCopyVariant=Disabled_SignalSpec  FilterICVariant=Disabled  IntegratorICVariant=InternalICs  ExternalResetVariant=Disabled  TRSumVariant=Passthrough  SumFdbkVariant=Disabled  SumVariant=Passthrough_I  TsampFilterVariant=InternalTs  TsampNgainVariant=Passthrough  TsampIntegralVariant=Disabled_SignalSpec  ExternalSaturationOutDataTypeStr=Inherit: Same as second input  DerivativeSourceVariant=Disabled
  Saturation : Saturate  UpperLimit=MPC_TILTMAX_AIR  LowerLimit=-MPC_TILTMAX_AIR
  Saturation1 : Saturate  UpperLimit=MPC_THR_MAX  LowerLimit=0
  Saturation2 : Saturate  UpperLimit=MPC_TILTMAX_AIR  LowerLimit=-MPC_TILTMAX_AIR
  Sum : Sum  Inputs=|+-
  Sum1 : Sum  Inputs=|+-
  Sum2 : Sum  Inputs=|+-
  Acc S.P : Outport
  wires:
  Setpoint velocity/1 -> Demux/1
  Demux/3 -> [SP_Vz]
  Demux1/3 -> [Vz]
  current velocity/1 -> Demux1/1
  Sum/1 -> Discrete-Time Integrator4/1, Gain/1
  Gain2/1 -> Add/3
  Discrete-Time Integrator4/1 -> Gain1/1
  Gain/1 -> Add/1
  Add/1 -> Saturation/1
  Add1/1 -> Display1/1, Saturation1/1
  Discrete-Time Integrator5/1 -> Gain4/1
  Gain5/1 -> Display3/1, Add1/3
  [Vz] -> LTI System2/1, Sum1/2  "Vz"
  [SP_Vz] -> Sum1/1  "s.p Vz"
  Saturation/1 -> Mux2/2
  Mux2/1 -> Display/1, Acc S.P/1
  Add2/1 -> Saturation2/1
  Gain6/1 -> Add2/1
  Gain8/1 -> Add2/3
  Sum2/1 -> Discrete-Time Integrator3/1, Gain6/1
  Demux/1 -> [SP_Vx]
  Demux/2 -> [SP_Vy]
  [SP_Vx] -> Sum2/1  "s.p Vx"
  [SP_Vy] -> Sum/1  "s.p Vy"
  Demux1/1 -> [Vx]
  [Vx] -> LTI System3/1, Sum2/2  "Vx"
  Demux1/2 -> [Vy]
  [Vy] -> LTI System1/1, Sum/2  "Vy"
  Saturation2/1 -> Mux2/1
  Saturation1/1 -> Mux2/3
  Discrete Derivative/1 -> Gain8/1
  Discrete Derivative1/1 -> Gain2/1
  Discrete Derivative2/1 -> Gain5/1
  Gain3/1 -> Display4/1, Add1/1
  Sum1/1 -> Discrete-Time Integrator5/1, Gain3/1
  Discrete-Time Integrator3/1 -> Gain7/1
  LTI System3/1 -> Discrete Derivative/1
  LTI System1/1 -> Discrete Derivative1/1
  Gain7/1 -> Add2/2
  Gain1/1 -> Add/2
  Gain4/1 -> Display2/1, Add1/2
  LTI System2/1 -> Discrete Derivative2/1

== system octocopter_control_flow/Inertial to Body/Norm3 ==
  In1 : Inport
  Dot Product : DotProduct  OutDataTypeStr=Inherit: Inherit via internal rule
  Math Function1 : Math  Operator=sqrt  SignedPower=on
  Out1 : Outport  VectorParamsAs1DForOutWhenUnconnected=off
  wires:
  Dot Product/1 -> Math Function1/1
  Math Function1/1 -> Out1/1
  In1/1 -> Dot Product/1, Dot Product/2

== system octocopter_control_flow/Inertial to Body/mavros attitude controller ==
  acc_cmd : Inport
  yaw : Inport  Port=2
  MATLAB Function : MATLAB Function  TreatAsAtomicUnit=on
  quat : Outport
  wires:
  MATLAB Function/1(quat) -> quat/1
  acc_cmd/1 -> MATLAB Function/1(vector_acc)
  yaw/1 -> MATLAB Function/2(yaw)

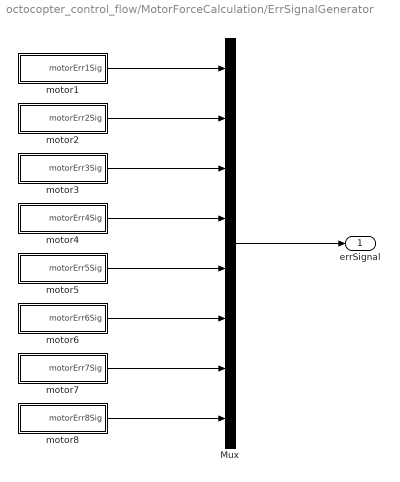
== system octocopter_control_flow/MotorForceCalculation/ErrSignalGenerator ==
  Mux : Mux  Inputs=8
  motor1 : Subsystem
  motor2 : Subsystem
  motor3 : Subsystem
  motor4 : Subsystem
  motor5 : Subsystem
  motor6 : Subsystem
  motor7 : Subsystem
  motor8 : Subsystem
  errSignal : Outport
  wires:
  Mux/1 -> errSignal/1
  motor1/1(motorErr1Sig) -> Mux/1
  motor2/1(motorErr2Sig) -> Mux/2
  motor3/1(motorErr3Sig) -> Mux/3
  motor4/1(motorErr4Sig) -> Mux/4
  motor5/1(motorErr5Sig) -> Mux/5
  motor6/1(motorErr6Sig) -> Mux/6
  motor7/1(motorErr7Sig) -> Mux/7
  motor8/1(motorErr8Sig) -> Mux/8

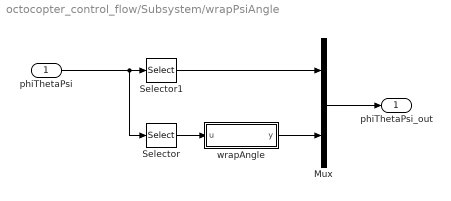
== system octocopter_control_flow/Subsystem/wrapPsiAngle ==
  phiThetaPsi : Inport
  Mux : Mux  Inputs=[2 1]
  Selector : Selector  InputPortWidth=3  IndexOptions=Index vector (dialog)  Indices=[3]  OutputSizes=1
  Selector1 : Selector  InputPortWidth=3  IndexOptions=Index vector (dialog)  Indices=[1 2]  OutputSizes=1
  wrapAngle : MATLAB Function  TreatAsAtomicUnit=on
  phiThetaPsi_out : Outport  VectorParamsAs1DForOutWhenUnconnected=off
  wires:
  Selector/1 -> wrapAngle/1(u)
  phiThetaPsi/1 -> Selector1/1, Selector/1
  wrapAngle/1(y) -> Mux/2
  Mux/1 -> phiThetaPsi_out/1
  Selector1/1 -> Mux/1

== system octocopter_control_flow/MotorForceCalculation/ErrSignalGenerator/motor1 ==
  note: err1Enable이 1이면 고장이 났다는 뜻이고,
      | 그러면 err1Enable =1 > 0 이니깐 motorErr1에서 나오는 신호를 출력하게 된다.
      | motorErr1은 initial value가 1, Final value가 0이다.
      | motorErr1Time이 5라면, 5초 전까지는 initial value를 주다가, 5초 이후에는 final Value를 준다.
      |
      |
      | err1Enable이 0이면 고장이 안 났다는 뜻이고,
      | 그러면 err1Enable =0 > 0 이니깐 constant 박스에 있는것을 신호로 출력하게 된다.
  Constant : Constant
  Constant1 : Constant  Value=err1Enable
  Switch : Switch  Criteria=u2 > Threshold  SaturateOnIntegerOverflow=off  InputSameDT=off
  motorErr1 : Step  Time=motorErr1Time  Before=1  After=0  SampleTime=0
  motorErr1Sig : Outport
  wires:
  Constant1/1 -> Switch/2
  Constant/1 -> Switch/3
  motorErr1/1 -> Switch/1
  Switch/1 -> motorErr1Sig/1

== system octocopter_control_flow/MotorForceCalculation/ErrSignalGenerator/motor2 ==
  Constant : Constant
  Constant1 : Constant  Value=err2Enable
  Switch : Switch  Criteria=u2 > Threshold  SaturateOnIntegerOverflow=off  InputSameDT=off
  motorErr2 : Step  Time=motorErr2Time  Before=1  After=0  SampleTime=0
  motorErr2Sig : Outport
  wires:
  Switch/1 -> motorErr2Sig/1
  motorErr2/1 -> Switch/1
  Constant/1 -> Switch/3
  Constant1/1 -> Switch/2

== system octocopter_control_flow/MotorForceCalculation/ErrSignalGenerator/motor3 ==
  Constant : Constant
  Constant1 : Constant  Value=err3Enable
  Switch : Switch  Criteria=u2 > Threshold  SaturateOnIntegerOverflow=off  InputSameDT=off
  motorErr3 : Step  Time=motorErr3Time  Before=1  After=0  SampleTime=0
  motorErr3Sig : Outport
  wires:
  Constant1/1 -> Switch/2
  Constant/1 -> Switch/3
  motorErr3/1 -> Switch/1
  Switch/1 -> motorErr3Sig/1

== system octocopter_control_flow/MotorForceCalculation/ErrSignalGenerator/motor4 ==
  Constant : Constant
  Constant1 : Constant  Value=err4Enable
  Switch : Switch  Criteria=u2 > Threshold  SaturateOnIntegerOverflow=off  InputSameDT=off
  motorErr4 : Step  Time=motorErr4Time  Before=1  After=0  SampleTime=0
  motorErr4Sig : Outport
  wires:
  Constant1/1 -> Switch/2
  Constant/1 -> Switch/3
  motorErr4/1 -> Switch/1
  Switch/1 -> motorErr4Sig/1

== system octocopter_control_flow/MotorForceCalculation/ErrSignalGenerator/motor5 ==
  Constant : Constant
  Constant1 : Constant  Value=err5Enable
  Switch : Switch  Criteria=u2 > Threshold  SaturateOnIntegerOverflow=off  InputSameDT=off
  motorErr5 : Step  Time=motorErr5Time  Before=1  After=0  SampleTime=0
  motorErr5Sig : Outport
  wires:
  Switch/1 -> motorErr5Sig/1
  motorErr5/1 -> Switch/1
  Constant/1 -> Switch/3
  Constant1/1 -> Switch/2

== system octocopter_control_flow/MotorForceCalculation/ErrSignalGenerator/motor6 ==
  Constant : Constant
  Constant1 : Constant  Value=err6Enable
  Switch : Switch  Criteria=u2 > Threshold  SaturateOnIntegerOverflow=off  InputSameDT=off
  motorErr6 : Step  Time=motorErr6Time  Before=1  After=0  SampleTime=0
  motorErr6Sig : Outport
  wires:
  Constant1/1 -> Switch/2
  Constant/1 -> Switch/3
  motorErr6/1 -> Switch/1
  Switch/1 -> motorErr6Sig/1

== system octocopter_control_flow/MotorForceCalculation/ErrSignalGenerator/motor7 ==
  Constant : Constant
  Constant1 : Constant  Value=err7Enable
  Switch : Switch  Criteria=u2 > Threshold  SaturateOnIntegerOverflow=off  InputSameDT=off
  motorErr7 : Step  Time=motorErr7Time  Before=1  After=0  SampleTime=0
  motorErr7Sig : Outport
  wires:
  Switch/1 -> motorErr7Sig/1
  motorErr7/1 -> Switch/1
  Constant/1 -> Switch/3
  Constant1/1 -> Switch/2

== system octocopter_control_flow/MotorForceCalculation/ErrSignalGenerator/motor8 ==
  Constant : Constant
  Constant1 : Constant  Value=err8Enable
  Switch : Switch  Criteria=u2 > Threshold  SaturateOnIntegerOverflow=off  InputSameDT=off
  motorErr8 : Step  Time=motorErr8Time  Before=1  After=0  SampleTime=0
  motorErr8Sig : Outport
  wires:
  Constant1/1 -> Switch/2
  Constant/1 -> Switch/3
  motorErr8/1 -> Switch/1
  Switch/1 -> motorErr8Sig/1

== matlab function octocopter_control_flow/Subsystem/wrapPsiAngle/wrapAngle ==
  data: u input; y output
function y = wrapAngle(u)
%#codegen
 % Wrap to [0 2*pi]
% y = u - 2*pi*floor(u/(2*pi));
y = u - 2*pi*floor((u+pi)/(2*pi)); % Wrap to [-pi pi]

== matlab function octocopter_control_flow/MotorForceCalculation/motorForceMomentCalc ==
  settings: updateMethod=DISCRETE
  data: desired_input output; omegaMotor input; FB output; Ct input; Cq input; MB output; C input
function [desired_input, FB,MB] = motorForceMomentCalc(omegaMotor,Ct,Cq,C)

% FB = [fx; fy; fz];
% MB = [mx; my; mz];


% persistent 변수 선언
persistent is_initialized FB_temp MB_temp;

% 초기화가 필요할 때만 실행
if isempty(is_initialized)
    % 임시 변수에 초기화
    FB_temp = zeros(3, 1);
    MB_temp = zeros(3, 1);
    is_initialized = true;
end

% C : 4by8
% omegaMotor : 8by1
% U = [fz;mx;my;mz] : 4by1
% disp('hihihihihihihihihihihhi')
% desired_input = u
desired_input = C * (abs(omegaMotor) .* abs(omegaMotor));
disp('omegaMotor = ')
disp(omegaMotor)
disp('omegaMotor.^2 = ')
disp(omegaMotor .* abs(omegaMotor))

FB_temp(1) = 0;
FB_temp(2) = 0;
FB_temp(3) = desired_input(1); % 추력 (Thrust)
MB_temp(1) = desired_input(2); % 롤 모멘트 (Roll moment)
MB_temp(2) = desired_input(3); % 피치 모멘트 (Pitch moment)
MB_temp(3) = desired_input(4); % 요 모멘트 (Yaw moment)

% 계산 결과를 출력 변수에 할당
FB = FB_temp;
MB = MB_temp;


end

== matlab function octocopter_control_flow/ControlMatrixAllocation Mixer/octo geometricCalc ==
  data: L1 input; C output; L2 input; L3 input; Ct input; Cq input
function C  = geometricCalc(L1,L2,L3,Ct,Cq)

% k= (1/sqrt(2));

% C : control matrix
% C+ : pseudo-inverse
% u* : pseudo input
% u : input

C = [ Ct,  Ct,  Ct,  Ct,  Ct,  Ct,  Ct,  Ct;
     -Ct*L1,  Ct*L1, -Ct*L1,  -Ct*L1,  Ct*L1, Ct*L1,  Ct*L1, -Ct*L1;
     -Ct*L3,  Ct*L3, -Ct*L2,  Ct*L3,  -Ct*L3, Ct*L2,  -Ct*L2,  Ct*L2;
      Cq,  Cq, -Cq, -Cq, -Cq, -Cq,  Cq,  Cq ];



% e = [ 0             -sin(alpha)     -cos(alpha);
%      -k*sin(alpha)  k*sin(alpha)    -cos(alpha);
%       sin(alpha)    0               -cos(alpha);
%      -k*sin(alpha)  -k*sin(alpha)   -cos(alpha);
%       0             sin(alpha)      -cos(alpha);
%       k*sin(alpha)  -k*sin(alpha)   -cos(alpha);
%      -sin(alpha)    0               -cos(alpha);
%       k*sin(alpha)  k*sin(alpha)    -cos(alpha)];
end

== matlab function octocopter_control_flow/MotorForceCalculation/ElementWiseMult ==
  data: omegaMotorSpeed input; omegaMotorSpeed_include_motor_fault_information output; errSignal input
function omegaMotorSpeed_include_motor_fault_information = fcn(omegaMotorSpeed,errSignal)

omegaMotorSpeed_include_motor_fault_information = omegaMotorSpeed.*errSignal;

== matlab function octocopter_control_flow/MATLAB Function ==
  data: M_B output; p_dot input; q_dot input; r_dot input; p input; q input; r input
function M_B = fcn(p_dot,q_dot,r_dot,p,q,r)


I_v = [7.46 0 0;0 1.53 0;0 0 8.89];

M_B = I_v * [p_dot;q_dot;r_dot] + cross([p;q;r] , I_v * [p;q;r]);
disp("M_B = ");
disp(size(M_B));

== matlab function octocopter_control_flow/Subsystem/modeling ==
  data: xyz input; VB input; phithetapsi input; OMEGAB input; x_dot output; y_dot output; z_dot output; u_dot output; v_dot output; w_dot output; phi_dot output; theta_dot output; psi_dot output; p_dot output; q_dot output; r_dot output; FB input; MB input
function [x_dot, y_dot, z_dot, u_dot, v_dot, w_dot, phi_dot, theta_dot, psi_dot, p_dot, q_dot, r_dot] = fcn(xyz,VB,phithetapsi,OMEGAB,FB,MB)



coder.extrinsic('RotMat');
coder.extrinsic('evalin');
coder.extrinsic('calculate_X_dot');


% persistent 변수 선언
persistent initialized;


% 초기화가 필요할 때만 실행
if isempty(initialized)
    % df_dx와 df_du를 미리 정의된 크기로 초기화
    x_dot = 0;
    y_dot = 0;
    z_dot = 0;
    u_dot = 0;
    v_dot = 0;
    w_dot = 0;
    phi_dot = 0;
    theta_dot = 0;
    psi_dot = 0;
    p_dot = 0;
    q_dot = 0;
    r_dot = 0;
    initialized = true; % 초기화 완료 표시
    disp('???? initialized.');
end


x=xyz(1);
y=xyz(2);
z=xyz(3);
u=VB(1);
v=VB(2);
w=VB(3);
phi = phithetapsi(1);
theta = phithetapsi(2);
psi = phithetapsi(3);
p = OMEGAB(1);
q = OMEGAB(2);
r = OMEGAB(3);
fx = FB(1);
fy = FB(2);
fz = FB(3);
mx = MB(1);
my = MB(2);
mz = MB(3);

[x_dot, y_dot, z_dot, u_dot, v_dot, w_dot,phi_dot,theta_dot,psi_dot,p_dot,q_dot,r_dot] = calculate_X_dot(x, y, z, u, v, w, phi, theta, psi, p, q, r,fx,fy,fz,mx,my,mz);



% x_dot = X_dot(1);
% y_dot = X_dot(2);
% z_dot = X_dot(3);
% u_dot = X_dot(4);
% v_dot = X_dot(5);
% w_dot = X_dot(6);
% phi_dot = X_dot(7);
% theta_dot = X_dot(8);
% psi_dot = X_dot(9);
% p_dot = X_dot(10);
% q_dot = X_dot(11);
% r_dot = X_dot(12);





end

== matlab function octocopter_control_flow/Inertial to Body/mavros attitude controller/MATLAB Function ==
  data: vector_acc input; quat output size=[1 4]; yaw input
function quat = fcn(vector_acc,yaw)

proj_xb_des = [cos(yaw) sin(yaw) 0];

zb_des = vector_acc / norm(vector_acc) ;
yb_des = cross(zb_des,proj_xb_des) / norm(cross(zb_des,proj_xb_des));
xb_des = cross(yb_des,zb_des) / norm(cross(yb_des,zb_des));

rotmat = [xb_des(1) yb_des(1) zb_des(1);xb_des(2) yb_des(2) zb_des(2);xb_des(3) yb_des(3) zb_des(3)];

quat = rotm2quat(rotmat);

== matlab function octocopter_control_flow/ControlMatrixAllocation Mixer/MATLAB Function ==
  settings: updateMethod=CONTINUOUS
  data: C input; motor_speed output; desired_u input
function motor_speed = fcn(C,desired_u)

% C : control matrix : 4by8
% C+ : pseudo-inverse 
% u* : pseudo input : desired input
% u : true input


% pseudo-inverse 계산
% C_pseudo_inverse = C' * inv(C * C');
C_pseudo_inverse = pinv(C); % pseudo-inverse 계산

% % 무어-펜로즈 역행렬의 크기 확인
% size_C_pseudo_inverse = size(C_pseudo_inverse);
% 
% % 결과 출력
% disp('C의 무어-펜로즈 역행렬 크기:');
% disp(size_C_pseudo_inverse);


% desired_u = C * (motor_speed^2)

motor_speed = C_pseudo_inverse * desired_u; % 각 모터에 필요한 출력 (속도 또는 추력)

== matlab function octocopter_control_flow/MotorForceCalculation/octo geometricCalc ==
  data: L1 input; C output; L2 input; L3 input; Ct input; Cq input; C_pseudo_inverse output
function [C,C_pseudo_inverse] = geometricCalc(L1,L2,L3,Ct,Cq)

% k= (1/sqrt(2));

% C : control matrix
% C+ : pseudo-inverse
% u* : pseudo input
% u : input
% u = C x u*

C = [ -Ct,  -Ct,  -Ct,  -Ct,  -Ct,  -Ct,  -Ct,  -Ct;
     -Ct*L1,  Ct*L1, -Ct*L1,  -Ct*L1,  Ct*L1, Ct*L1,  Ct*L1, -Ct*L1;
     Ct*L3,  -Ct*L3, Ct*L2,  -Ct*L3,  Ct*L3, -Ct*L2,  Ct*L2,  -Ct*L2;
      Cq,  Cq, -Cq, -Cq, -Cq, -Cq,  Cq,  Cq ];

C_pseudo_inverse = pinv(C)

% e = [ 0             -sin(alpha)     -cos(alpha);
%      -k*sin(alpha)  k*sin(alpha)    -cos(alpha);
%       sin(alpha)    0               -cos(alpha);
%      -k*sin(alpha)  -k*sin(alpha)   -cos(alpha);
%       0             sin(alpha)      -cos(alpha);
%       k*sin(alpha)  -k*sin(alpha)   -cos(alpha);
%      -sin(alpha)    0               -cos(alpha);
%       k*sin(alpha)  k*sin(alpha)    -cos(alpha)];
end
